simulink model "PathTrackingDriver"  (R2026b)
settings: Solver=ode4  StopTime=10  FixedStep=0.01
model workspace (MAT data in the model file):
  PathTrackingAntiWindupGain = 0.5
  PathTrackingBrakePressurePerAcceleration = 10000
  PathTrackingControlSampleTime = 0.01
  PathTrackingCrossTrackGain = 2
  PathTrackingHeadingGain = 1.2
  PathTrackingMaximumAcceleration = 8
  PathTrackingMaximumDeceleration = 8
  PathTrackingMaximumSteeringAngle = 0.5
  PathTrackingMaximumSteeringRate = 4
  PathTrackingMinimumSteeringSpeed = 1
  PathTrackingSpeedKi = 0.25
  PathTrackingSpeedKp = 0.8
  PathTrackingSteeringWheelRatio = 1
  PathTrackingWheelbase = 2
settings Model: DataDictionary=VehicleData.sldd  Creator=Xu Dingyi  LastModifiedBy=29358

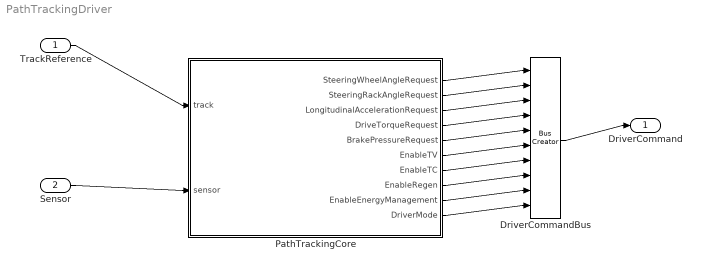
== system PathTrackingDriver ==
  TrackReference : Inport  OutDataTypeStr=Bus: TrackReferenceBus
  Sensor : Inport  Port=2  OutDataTypeStr=Bus: SensorBus
  DriverCommandBus : BusCreator  Inputs=10  OutDataTypeStr=Bus: DriverCommandBus
  PathTrackingCore : MATLAB Function  TreatAsAtomicUnit=on
  DriverCommand : Outport  OutDataTypeStr=Bus: DriverCommandBus
  wires:
  TrackReference/1 -> PathTrackingCore/1(track)
  Sensor/1 -> PathTrackingCore/2(sensor)
  PathTrackingCore/1(SteeringWheelAngleRequest) -> DriverCommandBus/1
  PathTrackingCore/2(SteeringRackAngleRequest) -> DriverCommandBus/2
  PathTrackingCore/3(LongitudinalAccelerationRequest) -> DriverCommandBus/3
  PathTrackingCore/4(DriveTorqueRequest) -> DriverCommandBus/4
  PathTrackingCore/5(BrakePressureRequest) -> DriverCommandBus/5
  PathTrackingCore/6(EnableTV) -> DriverCommandBus/6
  PathTrackingCore/7(EnableTC) -> DriverCommandBus/7
  PathTrackingCore/8(EnableRegen) -> DriverCommandBus/8
  PathTrackingCore/9(EnableEnergyManagement) -> DriverCommandBus/9
  PathTrackingCore/10(DriverMode) -> DriverCommandBus/10
  DriverCommandBus/1 -> DriverCommand/1

== matlab function PathTrackingDriver/PathTrackingCore ==
  data: track input; SteeringWheelAngleRequest output; sensor input; SteeringRackAngleRequest output; LongitudinalAccelerationRequest output; DriveTorqueRequest output; BrakePressureRequest output; EnableTV output; EnableTC output; EnableRegen output; EnableEnergyManagement output; DriverMode output; PathTrackingControlSampleTime parameter; PathTrackingWheelbase parameter; PathTrackingHeadingGain parameter; PathTrackingCrossTrackGain parameter; PathTrackingMinimumSteeringSpeed parameter; PathTrackingMaximumSteeringAngle parameter; PathTrackingMaximumSteeringRate parameter; PathTrackingSteeringWheelRatio parameter; PathTrackingSpeedKp parameter; PathTrackingSpeedKi parameter; PathTrackingAntiWindupGain parameter; PathTrackingMaximumAcceleration parameter; PathTrackingMaximumDeceleration parameter; PathTrackingBrakePressurePerAcceleration parameter
function [SteeringWheelAngleRequest, SteeringRackAngleRequest, ...
    LongitudinalAccelerationRequest, DriveTorqueRequest, ...
    BrakePressureRequest, EnableTV, EnableTC, EnableRegen, ...
    EnableEnergyManagement, DriverMode] = fcn(track, sensor, PathTrackingControlSampleTime, PathTrackingWheelbase, PathTrackingHeadingGain, PathTrackingCrossTrackGain, PathTrackingMinimumSteeringSpeed, PathTrackingMaximumSteeringAngle, PathTrackingMaximumSteeringRate, PathTrackingSteeringWheelRatio, PathTrackingSpeedKp, PathTrackingSpeedKi, PathTrackingAntiWindupGain, PathTrackingMaximumAcceleration, PathTrackingMaximumDeceleration, PathTrackingBrakePressurePerAcceleration)
%FSAEPathTrackingPATHTRACKINGCORE Discrete Stanley-style lateral and PI speed control.
%   Sensor is used instead of VehicleState, so the production driver model
%   does not depend directly on plant truth.

persistent speedIntegrator previousSteering
if isempty(speedIntegrator)
    speedIntegrator = 0;
    previousSteering = 0;
end

SteeringWheelAngleRequest = 0;
SteeringRackAngleRequest = 0;
LongitudinalAccelerationRequest = 0;
DriveTorqueRequest = 0;
BrakePressureRequest = 0;
EnableTV = false;
EnableTC = false;
EnableRegen = true;
EnableEnergyManagement = false;
DriverMode = uint8(0);

if ~track.Valid || ~sensor.PoseValid
    return
end
DriverMode = uint8(2);

deltaX = sensor.PositionX - track.ReferenceX;
deltaY = sensor.PositionY - track.ReferenceY;
lateralError = -deltaX * sin(track.ReferenceHeading) + ...
    deltaY * cos(track.ReferenceHeading);
headingError = atan2(sin(track.ReferenceHeading - sensor.Heading), ...
    cos(track.ReferenceHeading - sensor.Heading));
speedForSteering = max(abs(sensor.LongitudinalSpeed), PathTrackingMinimumSteeringSpeed);
curvatureFeedForward = atan(PathTrackingWheelbase * track.ReferenceCurvature);
feedbackSteering = PathTrackingHeadingGain * headingError - ...
    atan2(PathTrackingCrossTrackGain * lateralError, speedForSteering);
requestedSteering = curvatureFeedForward + feedbackSteering;
requestedSteering = min(PathTrackingMaximumSteeringAngle, ...
    max(-PathTrackingMaximumSteeringAngle, requestedSteering));
steeringRateLimit = PathTrackingMaximumSteeringRate * PathTrackingControlSampleTime;
SteeringRackAngleRequest = previousSteering + min(steeringRateLimit, ...
    max(-steeringRateLimit, requestedSteering - previousSteering));
previousSteering = SteeringRackAngleRequest;
SteeringWheelAngleRequest = PathTrackingSteeringWheelRatio * SteeringRackAngleRequest;

speedError = track.ReferenceSpeed - sensor.LongitudinalSpeed;
unsaturatedAcceleration = PathTrackingSpeedKp * speedError + speedIntegrator;
LongitudinalAccelerationRequest = min(PathTrackingMaximumAcceleration, ...
    max(-PathTrackingMaximumDeceleration, unsaturatedAcceleration));
integratorError = LongitudinalAccelerationRequest - unsaturatedAcceleration;
speedIntegrator = speedIntegrator + PathTrackingSpeedKi * speedError * ...
    PathTrackingControlSampleTime + PathTrackingAntiWindupGain * integratorError * ...
    PathTrackingControlSampleTime;

% The PathTracking baseline uses the acceleration request as the controller contract;
% the controller converts it to motor and regenerative torque.  The brake
% pressure field is kept explicit but disabled until a pressure map exists.
BrakePressureRequest = max(0, -LongitudinalAccelerationRequest) * ...
    PathTrackingBrakePressurePerAcceleration;
EnableTC = true;
end
